simulink model "tag_vbap"  (R2022a)
settings: Solver=VariableStepAuto  StartTime=0.0  StopTime=10.0  RelTol=1e-3
settings Model: Creator=mheubach  LastModifiedBy=mheubach

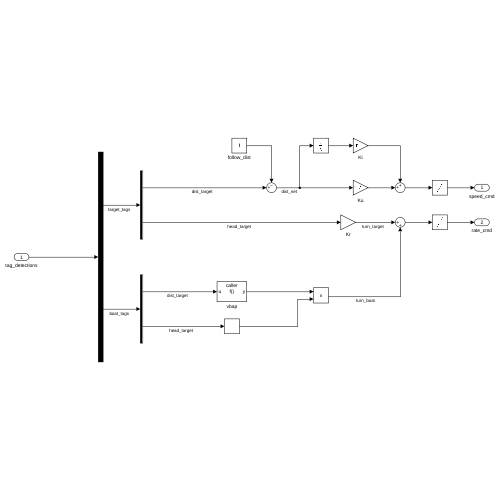
[thumbnail: Simulink's stored preview of the top-level diagram]
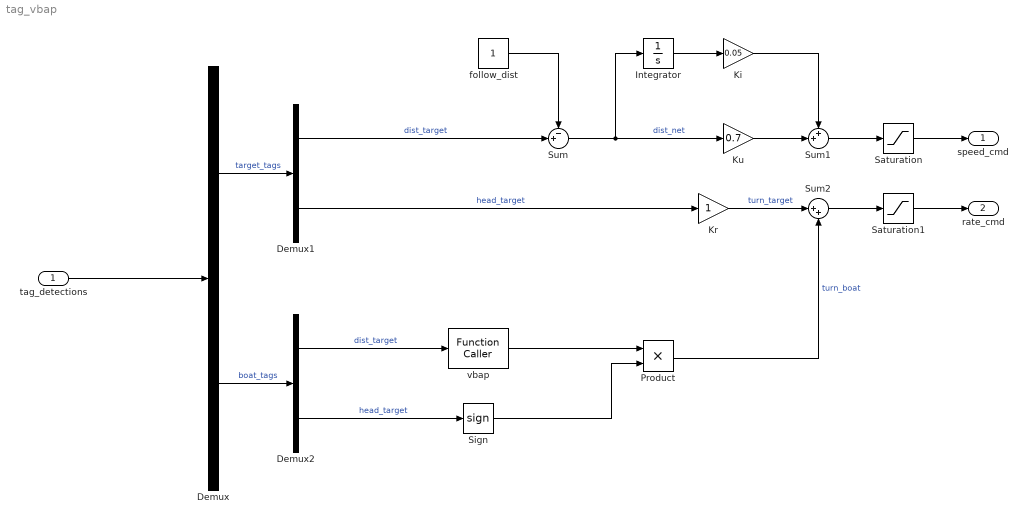
== system tag_vbap ==
  tag_detections : Inport
  Demux : Demux  Outputs=2
  Demux1 : Demux  Outputs=2
  Demux2 : Demux  Outputs=2
  Integrator : Integrator
  Ki : Gain  Gain=0.05
  Kr : Gain
  Ku : Gain  Gain=0.7
  Product : Product
  Saturation : Saturate
  Saturation1 : Saturate
  Sign : Signum
  Sum : Sum  Inputs=-+|
  Sum1 : Sum  Inputs=++|
  Sum2 : Sum  Inputs=|++
  follow_dist : Constant
  vbap : FunctionCaller  FunctionPrototype=y = f(u)  InputArgumentSpecifications=<Enter example>  OutputArgumentSpecifications=<Enter example>
  speed_cmd : Outport
  rate_cmd : Outport  Port=2
  wires:
  tag_detections/1 -> Demux/1
  Demux/2 -> Demux2/1  "boat_tags"
  Demux/1 -> Demux1/1  "target_tags"
  Demux1/1 -> Sum/2  "dist_target"
  follow_dist/1 -> Sum/1
  Sum/1 -> Ku/1, Integrator/1  "dist_net"
  Integrator/1 -> Ki/1
  Ki/1 -> Sum1/1
  Ku/1 -> Sum1/2
  Sum1/1 -> Saturation/1
  Saturation/1 -> speed_cmd/1
  Demux1/2 -> Kr/1  "head_target"
  Demux2/2 -> Sign/1  "head_target"
  Demux2/1 -> vbap/1  "dist_target"
  Sign/1 -> Product/2
  vbap/1 -> Product/1
  Product/1 -> Sum2/2  "turn_boat"
  Kr/1 -> Sum2/1  "turn_target"
  Sum2/1 -> Saturation1/1
  Saturation1/1 -> rate_cmd/1
